simulink model "Energy"  (R2024b)
settings: Solver=ode1  StartTime=0.0  StopTime=955800  FixedStep=1  RelTol=1e-3
(part 2 of 3)

== matlab function Energy/工况生成器 ==
  data: t input; P_out output
function P_out = fcn(t)
%% 工况生成函数2
%% 输入: t - 仿真时间 (s)
%% 输出: P_out - 功率 (kW)

%% ===== 工况数据 =====
% 功率点 (kW)
P_table = [64.039, 57.95, 72.892, 53.239, 371.167, 81.182, 152.606, ...
           55.814, 52.287, 87.468, 57.663, 57.95, 64.502];

% 持续时间 (s) = 小时 × 3600
T_duration = [3, 112, 5, 6, 0.2, 8, 8, 3, 0.3, 1, 4, 112, 3] * 3600;

%% ===== 累计时间断点 =====
T_bp = [0, 10800, 414000, 432000, 453600, 454320, 483120, 511920, ...
        522720, 523800, 527400, 541800, 945000, 955800];

%% ===== 根据时间查找功率 =====
n = 13;
P_out = P_table(n);  % 默认最后一个

for k = 1:n
    if t >= T_bp(k) && t < T_bp(k+1)
        P_out = P_table(k);
        break;
    end
end

end

== matlab function Energy/Subsystem6/DCDC1_2 ==
  data: V_out input; I_in input; V_in input; I_out output
function I_out = fcn(V_out,I_in, V_in)
%% DCDC模型 - 输入电流计算输出电流
%% 输入:
%%   I_in  - 输入电流 (A)
%%   V_in  - 输入电压 (V)
%%   V_out - 输出电压 (V)
%% 输出:
%%   I_out - 输出电流 (A)

%% ===== 效率MAP表 =====
% 输入电压断点 (V)
V_bp = [160, 180, 200, 220, 240, 260, 280];

% 输入电流断点 (A)
I_bp = [0, 20, 40, 60, 80, 100, 120, 140, 160, 180, 200];

% 效率表 (%)，行=电流，列=电压
Eta_map = [
    86, 86, 86, 86, 86, 86, 86;
    88, 88, 87, 87, 87, 87, 86;
    92, 91, 91, 90, 89, 88, 87;
    94, 93, 93, 92, 91, 90, 88;
    94.5, 94, 94, 93, 92, 91, 89;
    95, 94.5, 94, 93.5, 93, 91, 90;
    95, 94.5, 94.5, 94, 93, 92, 91;
    95, 95, 94.5, 94, 93.5, 93, 91;
    95, 95, 94.5, 94, 93, 92, 91;
    95, 94.5, 94.5, 93, 92, 91, 91;
    95, 94.5, 94, 92, 91, 91, 91
] / 100;

%% ===== 输入限幅 =====
V_in_clamp = max(160, min(280, V_in));
I_in_clamp = max(0, min(200, I_in));

%% ===== 查表获取效率 =====
% 找电压区间
nV = 7;
jV = 1;
for j = 1:nV-1
    if V_in_clamp >= V_bp(j) && V_in_clamp <= V_bp(j+1)
        jV = j;
        break;
    end
end
if V_in_clamp >= V_bp(nV)
    jV = nV - 1;
end
tV = (V_in_clamp - V_bp(jV)) / (V_bp(jV+1) - V_bp(jV));

% 找电流区间
nI = 11;
iI = 1;
for i = 1:nI-1
    if I_in_clamp >= I_bp(i) && I_in_clamp <= I_bp(i+1)
        iI = i;
        break;
    end
end
if I_in_clamp >= I_bp(nI)
    iI = nI - 1;
end
tI = (I_in_clamp - I_bp(iI)) / (I_bp(iI+1) - I_bp(iI));

% 双线性插值
eta_11 = Eta_map(iI, jV);
eta_12 = Eta_map(iI, jV+1);
eta_21 = Eta_map(iI+1, jV);
eta_22 = Eta_map(iI+1, jV+1);

eta_1 = eta_11 + tV * (eta_12 - eta_11);
eta_2 = eta_21 + tV * (eta_22 - eta_21);
eta = eta_1 + tI * (eta_2 - eta_1);

%% ===== 计算输出电流 =====
P_in = V_in * I_in;
P_out = P_in * eta;
V_out_safe = max(V_out, 1);
I_out = P_out / V_out_safe;

end

== matlab function Energy/Subsystem/目标输出功率 ==
  data: P_target input; dt input; P_out output
function P_out = fcn(P_target, dt)
%% 燃料电池预热控制器 - 带热机跳过功能
%% 输入:
%%   P_target - 目标功率 (kW)
%%   dt       - 采样时间 (s)
%% 输出:
%%   P_out    - 输出功率 (kW)

%% ===== 参数设置 =====
T_warmup = 1800;       % 预热时间 30分钟
P_warmup = 5;          % 预热功率上限 5kW
T_hot_keep = 18000;    % 热机保持时间 5小时 = 5*3600s

%% ===== 状态变量 =====
persistent timer_run timer_stop is_running is_hot
if isempty(timer_run)
    timer_run = 0;      % 运行计时器
    timer_stop = 0;     % 停机计时器
    is_running = 0;     % 运行状态
    is_hot = 0;         % 热机状态：0=冷机，1=已热机
end

%% ===== 状态机逻辑 =====
if P_target > 0
    % 启动/运行中
    if is_running == 0
        % 刚启动
        is_running = 1;
        timer_run = 0;
        
        % 判断是否需要热机
        if is_hot == 1 && timer_stop <= T_hot_keep
            % 停机5小时内，跳过热机
            timer_run = T_warmup + 1;  % 直接跳过热机阶段
        else
            % 冷机或停机超过5小时，需要热机
            timer_run = 0;
        end
    end
    
    timer_run = timer_run + dt;
    timer_stop = 0;  % 清空停机计时
    
    % 完成热机后标记
    if timer_run > T_warmup
        is_hot = 1;
    end
else
    % 停机
    if is_running == 1
        % 刚停机
        is_running = 0;
        timer_stop = 0;
    end
    
    timer_stop = timer_stop + dt;
    timer_run = 0;
    
    % 停机超过5小时，热机状态清除
    if timer_stop > T_hot_keep
        is_hot = 0;
    end
end

%% ===== 功率选择 =====
if P_target <= 0
    P_out = 0;
elseif timer_run <= T_warmup
    % 热机阶段，限制最大5kW
    P_out = min(P_target, P_warmup);
else
    % 热机完成，输出等于输入
    P_out = P_target;
end

end

== matlab function Energy/Subsystem/DCDC1_1 ==
  data: P_out input; V_out input; I_out output; V_in input; I_in output
function [I_out, I_in] = fcn(P_out, V_out, V_in)
%% DCDC模型 - 输出功率反算输入电流
%% 输入:
%%   P_out - 输出功率 (W)
%%   V_out - 输出电压 (V)
%%   V_in  - 输入电压 (V)
%% 输出:
%%   I_out - 输出电流 (A)
%%   I_in  - 输入电流 (A)

%% ===== 效率MAP表 =====
% 输入电压断点 (V)
V_bp = [160, 180, 200, 220, 240, 260, 280];

% 输入电流断点 (A)
I_bp = [0, 20, 40, 60, 80, 100, 120, 140, 160, 180, 200];

% 效率表 (%)，行=电流，列=电压
Eta_map = [
    86, 86, 86, 86, 86, 86, 86;
    88, 88, 87, 87, 87, 87, 86;
    92, 91, 91, 90, 89, 88, 87;
    94, 93, 93, 92, 91, 90, 88;
    94.5, 94, 94, 93, 92, 91, 89;
    95, 94.5, 94, 93.5, 93, 91, 90;
    95, 94.5, 94.5, 94, 93, 92, 91;
    95, 95, 94.5, 94, 93.5, 93, 91;
    95, 95, 94.5, 94, 93, 92, 91;
    95, 94.5, 94.5, 93, 92, 91, 91;
    95, 94.5, 94, 92, 91, 91, 91
] / 100;

%% ===== 输出电流（直接计算） =====
V_out_safe = max(V_out, 1);
I_out = 1000*P_out / V_out_safe;

%% ===== 迭代求输入电流 =====
V_in_clamp = max(160, min(280, V_in));
V_in_safe = max(V_in, 1);

% 初始估计效率
eta = 0.94;

% 迭代3次足够收敛
for iter = 1:3
    % 根据效率计算输入功率和电流
    P_in = 1000*P_out / eta;
    I_in_est = P_in / V_in_safe;
    I_in_clamp = max(0, min(200, I_in_est));
    
    % 查表获取新效率
    eta = lookup_eta(V_in_clamp, I_in_clamp, V_bp, I_bp, Eta_map);
end

%% ===== 最终输入电流 =====
P_in = 1000*P_out / eta;
I_in = P_in / V_in_safe;

end

%% ===== 效率查表函数 =====
function eta = lookup_eta(V_in, I_in, V_bp, I_bp, Eta_map)
    % 找电压区间
    nV = 7;
    jV = 1;
    for j = 1:nV-1
        if V_in >= V_bp(j) && V_in <= V_bp(j+1)
            jV = j;
            break;
        end
    end
    if V_in >= V_bp(nV)
        jV = nV - 1;
    end
    tV = (V_in - V_bp(jV)) / (V_bp(jV+1) - V_bp(jV));
    
    % 找电流区间
    nI = 11;
    iI = 1;
    for i = 1:nI-1
        if I_in >= I_bp(i) && I_in <= I_bp(i+1)
            iI = i;
            break;
        end
    end
    if I_in >= I_bp(nI)
        iI = nI - 1;
    end
    tI = (I_in - I_bp(iI)) / (I_bp(iI+1) - I_bp(iI));
    
    % 双线性插值
    eta_11 = Eta_map(iI, jV);
    eta_12 = Eta_map(iI, jV+1);
    eta_21 = Eta_map(iI+1, jV);
    eta_22 = Eta_map(iI+1, jV+1);
    
    eta_1 = eta_11 + tV * (eta_12 - eta_11);
    eta_2 = eta_21 + tV * (eta_22 - eta_21);
    eta = eta_1 + tI * (eta_2 - eta_1);
end

== matlab function Energy/Subsystem/输出电流加载限制 ==
  data: I_target input; I_current input; I_out output; dt input
function I_out = fcn(I_target,I_current,  dt)
%% 电流斜坡控制器 - 反馈版
%% 输入:
%%   I_current - 当前电流 (A)，从输出反馈
%%   I_target  - 目标电流 (A) 
%%   dt        - 采样时间 (s)
%% 输出:
%%   I_out     - 输出电流 (A)

%% ===== 参数设置 =====
rate_up = 1;    % 上升速率 1A/s
rate_down = 2;  % 下降速率 2A/s

%% ===== 斜坡控制 =====
delta = I_target - I_current;

if delta > 0
    % 目标 > 当前，每秒+1A
    I_out = I_current + rate_up * dt;
    if I_out > I_target
        I_out = I_target;
    end
elseif delta < 0
    % 目标 < 当前，每秒-2A
    I_out = I_current - rate_down * dt;
    if I_out < I_target
        I_out = I_target;
    end
else
    I_out = I_current;
end

%% ===== 输出限幅 =====
I_out = max(0, I_out);

end

== matlab function Energy/Subsystem/DCDC1_2 ==
  data: V_out input; I_in input; V_in input; I_out output
function I_out = fcn(V_out,I_in, V_in)
%% DCDC模型 - 输入电流计算输出电流
%% 输入:
%%   I_in  - 输入电流 (A)
%%   V_in  - 输入电压 (V)
%%   V_out - 输出电压 (V)
%% 输出:
%%   I_out - 输出电流 (A)

%% ===== 效率MAP表 =====
% 输入电压断点 (V)
V_bp = [160, 180, 200, 220, 240, 260, 280];

% 输入电流断点 (A)
I_bp = [0, 20, 40, 60, 80, 100, 120, 140, 160, 180, 200];

% 效率表 (%)，行=电流，列=电压
Eta_map = [
    86, 86, 86, 86, 86, 86, 86;
    88, 88, 87, 87, 87, 87, 86;
    92, 91, 91, 90, 89, 88, 87;
    94, 93, 93, 92, 91, 90, 88;
    94.5, 94, 94, 93, 92, 91, 89;
    95, 94.5, 94, 93.5, 93, 91, 90;
    95, 94.5, 94.5, 94, 93, 92, 91;
    95, 95, 94.5, 94, 93.5, 93, 91;
    95, 95, 94.5, 94, 93, 92, 91;
    95, 94.5, 94.5, 93, 92, 91, 91;
    95, 94.5, 94, 92, 91, 91, 91
] / 100;

%% ===== 输入限幅 =====
V_in_clamp = max(160, min(280, V_in));
I_in_clamp = max(0, min(200, I_in));

%% ===== 查表获取效率 =====
% 找电压区间
nV = 7;
jV = 1;
for j = 1:nV-1
    if V_in_clamp >= V_bp(j) && V_in_clamp <= V_bp(j+1)
        jV = j;
        break;
    end
end
if V_in_clamp >= V_bp(nV)
    jV = nV - 1;
end
tV = (V_in_clamp - V_bp(jV)) / (V_bp(jV+1) - V_bp(jV));

% 找电流区间
nI = 11;
iI = 1;
for i = 1:nI-1
    if I_in_clamp >= I_bp(i) && I_in_clamp <= I_bp(i+1)
        iI = i;
        break;
    end
end
if I_in_clamp >= I_bp(nI)
    iI = nI - 1;
end
tI = (I_in_clamp - I_bp(iI)) / (I_bp(iI+1) - I_bp(iI));

% 双线性插值
eta_11 = Eta_map(iI, jV);
eta_12 = Eta_map(iI, jV+1);
eta_21 = Eta_map(iI+1, jV);
eta_22 = Eta_map(iI+1, jV+1);

eta_1 = eta_11 + tV * (eta_12 - eta_11);
eta_2 = eta_21 + tV * (eta_22 - eta_21);
eta = eta_1 + tI * (eta_2 - eta_1);

%% ===== 计算输出电流 =====
P_in = V_in * I_in;
P_out = P_in * eta;
V_out_safe = max(V_out, 1);
I_out = P_out / V_out_safe;

end

== matlab function Energy/Subsystem6/目标输出功率 ==
  data: P_target input; dt input; P_out output
function P_out = fcn(P_target, dt)
%% 燃料电池预热控制器 - 带热机跳过功能
%% 输入:
%%   P_target - 目标功率 (kW)
%%   dt       - 采样时间 (s)
%% 输出:
%%   P_out    - 输出功率 (kW)

%% ===== 参数设置 =====
T_warmup = 1800;       % 预热时间 30分钟
P_warmup = 5;          % 预热功率上限 5kW
T_hot_keep = 18000;    % 热机保持时间 5小时 = 5*3600s

%% ===== 状态变量 =====
persistent timer_run timer_stop is_running is_hot
if isempty(timer_run)
    timer_run = 0;      % 运行计时器
    timer_stop = 0;     % 停机计时器
    is_running = 0;     % 运行状态
    is_hot = 0;         % 热机状态：0=冷机，1=已热机
end

%% ===== 状态机逻辑 =====
if P_target > 0
    % 启动/运行中
    if is_running == 0
        % 刚启动
        is_running = 1;
        timer_run = 0;
        
        % 判断是否需要热机
        if is_hot == 1 && timer_stop <= T_hot_keep
            % 停机5小时内，跳过热机
            timer_run = T_warmup + 1;  % 直接跳过热机阶段
        else
            % 冷机或停机超过5小时，需要热机
            timer_run = 0;
        end
    end
    
    timer_run = timer_run + dt;
    timer_stop = 0;  % 清空停机计时
    
    % 完成热机后标记
    if timer_run > T_warmup
        is_hot = 1;
    end
else
    % 停机
    if is_running == 1
        % 刚停机
        is_running = 0;
        timer_stop = 0;
    end
    
    timer_stop = timer_stop + dt;
    timer_run = 0;
    
    % 停机超过5小时，热机状态清除
    if timer_stop > T_hot_keep
        is_hot = 0;
    end
end

%% ===== 功率选择 =====
if P_target <= 0
    P_out = 0;
elseif timer_run <= T_warmup
    % 热机阶段，限制最大5kW
    P_out = min(P_target, P_warmup);
else
    % 热机完成，输出等于输入
    P_out = P_target;
end

end

== matlab function Energy/240kW功率分配 ==
  data: V_battery input; SOC input; P_battery input; P1 output; P2 output; P3 output; P4 output; P5 output; P6 output; P7 output; P8 output; P_fuelcell input; dt input
function [P1, P2, P3, P4, P5, P6, P7, P8] = fcn(V_battery, SOC, P_battery, P_fuelcell, dt)
%% 能量管理控制器 - 不停机策略
%% 挡位: 0(仅P_load=0), 50, 65, 85, 120 kW
%% 
%% 核心规则：
%% 1. 只有P_load=0才允许停机，否则至少保持1档运行
%% 2. SOC硬保护：0.5-0.9，超限立即响应
%% 3. 正常模式：滞回切换 + 冷却时间

%% ===== SOC硬保护阈值 =====
SOC_max = 0.9;
SOC_min = 0.5;
SOC_discharge_stop = 0.65;
SOC_charge_stop = 0.7;

%% ===== 挡位功率 (kW) =====
% 0档=0, 1档=50, 2档=65, 3档=85, 4档=120
Gear_power = [0, 50, 65, 85, 120];

%% ===== 挡位切换阈值 (kW) =====
% 主力挡位2档(65kW)覆盖55-75kW
Gear_up = [1, 55, 75, 100];       % 0→1, 1→2, 2→3, 3→4
Gear_down = [0, 48, 68, 88];      % 1→0(仅P=0), 2→1, 3→2, 4→3

%% ===== 冷却时间 =====
T_cooldown = 120;

%% ===== 过载阈值 =====
P_overload = 150;

%% ===== 状态变量 =====
persistent gear_state discharge_mode charge_mode cooldown_timer
if isempty(gear_state)
    gear_state = 2;  % 初始65kW挡
    discharge_mode = 0;
    charge_mode = 0;
    cooldown_timer = 0;
end

%% ===== 更新冷却计时器 =====
if cooldown_timer > 0
    cooldown_timer = cooldown_timer - dt;
end

%% ===== 计算负载功率 (kW) =====
P_load = P_fuelcell + P_battery;
P_load = max(0, P_load);

%% ===== 停机判断：仅当P_load=0 =====
if P_load < 0.1
    % 完全无负载才停机
    gear_state = 0;
    P1 = 0; P2 = 0; P3 = 0; P4 = 0;
    P5 = 0; P6 = 0; P7 = 0; P8 = 0;
    
elseif P_load > P_overload
    %% ===== 过载保护 =====
    gear_state = 4;
    P1 = 30; P2 = 30; P3 = 30; P4 = 30;
    P5 = 0; P6 = 0; P7 = 0; P8 = 0;
    
else
    %% ===== 从停机恢复 =====
    if gear_state == 0
        gear_state = 2;  % 恢复到主力档位
        cooldown_timer = T_cooldown;
    end
    
    %% ===== SOC保护模式滞回更新 =====
    if SOC > SOC_max
        discharge_mode = 1;
    elseif SOC <= SOC_discharge_stop
        discharge_mode = 0;
    end
    
    if SOC < SOC_min
        charge_mode = 1;
    elseif SOC >= SOC_charge_stop
        charge_mode = 0;
    end
    
    %% ===== SOC硬保护（立即响应）=====
    if discharge_mode == 1
        % SOC > 0.9：降档让电池放电
        if P_battery <= 0
            gear_state = gear_state - 1;
            % 最低降到1档，不停机！
            if gear_state < 1
                gear_state = 1;
            end
        end
        
    elseif charge_mode == 1
        % SOC < 0.5：升档让电池充电
        if P_battery >= 0
            gear_state = gear_state + 1;
            if gear_state > 4
                gear_state = 4;
            end
        end
        
    else
        %% ===== 正常模式：滞回切换 =====
        if cooldown_timer <= 0
            need_change = 0;
            
            % 注意：不会降到0档（除非P_load=0已在前面处理）
            if gear_state == 1
                if P_load > Gear_up(2)
                    gear_state = 2;
                    need_change = 1;
                end
            elseif gear_state == 2
                if P_load < Gear_down(2)
                    gear_state = 1;
                    need_change = 1;
                elseif P_load > Gear_up(3)
                    gear_state = 3;
                    need_change = 1;
                end
            elseif gear_state == 3
                if P_load < Gear_down(3)
                    gear_state = 2;
                    need_change = 1;
                elseif P_load > Gear_up(4)
                    gear_state = 4;
                    need_change = 1;
                end
            elseif gear_state == 4
                if P_load < Gear_down(4)
                    gear_state = 3;
                    need_change = 1;
                end
            end
            
            if need_change == 1
                cooldown_timer = T_cooldown;
            end
        end
    end
    
    %% ===== 按挡位分配功率 =====
    if gear_state == 1
        P1 = 12.5; P2 = 12.5; P3 = 12.5; P4 = 12.5;  % 50kW
    elseif gear_state == 2
        P1 = 16.25; P2 = 16.25; P3 = 16.25; P4 = 16.25;  % 65kW
    elseif gear_state == 3
        P1 = 21.25; P2 = 21.25; P3 = 21.25; P4 = 21.25;  % 85kW
    else
        P1 = 30; P2 = 30; P3 = 30; P4 = 30;  % 120kW
    end
    P5 = 0; P6 = 0; P7 = 0; P8 = 0;
end

end

== matlab function Energy/Subsystem6/输出电流加载限制 ==
  data: I_target input; I_current input; I_out output; dt input
function I_out = fcn(I_target,I_current,  dt)
%% 电流斜坡控制器 - 反馈版
%% 输入:
%%   I_current - 当前电流 (A)，从输出反馈
%%   I_target  - 目标电流 (A) 
%%   dt        - 采样时间 (s)
%% 输出:
%%   I_out     - 输出电流 (A)

%% ===== 参数设置 =====
rate_up = 1;    % 上升速率 1A/s
rate_down = 2;  % 下降速率 2A/s

%% ===== 斜坡控制 =====
delta = I_target - I_current;

if delta > 0
    % 目标 > 当前，每秒+1A
    I_out = I_current + rate_up * dt;
    if I_out > I_target
        I_out = I_target;
    end
elseif delta < 0
    % 目标 < 当前，每秒-2A
    I_out = I_current - rate_down * dt;
    if I_out < I_target
        I_out = I_target;
    end
else
    I_out = I_current;
end

%% ===== 输出限幅 =====
I_out = max(0, I_out);

end

== matlab function Energy/Subsystem7/32kW燃料电池 ==
  data: I_in input; V output
function V = fcn(I_in)
%% 燃料电池模型 - 极化曲线
%% 输入: I_in - 输入电流 (A)
%% 输出: V    - 输出电压 (V)

%% ===== 极化曲线数据 =====
I_table = [0, 16.77, 31.67, 48.13, 64.92, 80.76, 98.06, 115.48, 132.58, 150.51, 170.44, 186.07];
V_table = [248.1, 218.42, 212.82, 207.8, 205, 202.68, 200, 197.8, 196.44, 194.26, 192.66, 191.2];

%% ===== 电流限幅 =====
I_max = 186.07;
I = max(0, min(I_in, I_max));

%% ===== 根据电流查找电压 =====
V = V_table(1);  % 初始化
n = 12;

for k = 1:n-1
    if I >= I_table(k) && I <= I_table(k+1)
        t = (I - I_table(k)) / (I_table(k+1) - I_table(k));
        V = V_table(k) + t * (V_table(k+1) - V_table(k));
        break;
    end
end

if I >= I_table(n)
    V = V_table(n);
end

end

== matlab function Energy/Subsystem/32kW燃料电池 ==
  data: I_in input; V output
function V = fcn(I_in)
%% 燃料电池模型 - 极化曲线
%% 输入: I_in - 输入电流 (A)
%% 输出: V    - 输出电压 (V)

%% ===== 极化曲线数据 =====
I_table = [0, 16.77, 31.67, 48.13, 64.92, 80.76, 98.06, 115.48, 132.58, 150.51, 170.44, 186.07];
V_table = [248.1, 218.42, 212.82, 207.8, 205, 202.68, 200, 197.8, 196.44, 194.26, 192.66, 191.2];

%% ===== 电流限幅 =====
I_max = 186.07;
I = max(0, min(I_in, I_max));

%% ===== 根据电流查找电压 =====
V = V_table(1);  % 初始化
n = 12;

for k = 1:n-1
    if I >= I_table(k) && I <= I_table(k+1)
        t = (I - I_table(k)) / (I_table(k+1) - I_table(k));
        V = V_table(k) + t * (V_table(k+1) - V_table(k));
        break;
    end
end

if I >= I_table(n)
    V = V_table(n);
end

end

== matlab function Energy/Subsystem7/DCDC1_1 ==
  data: P_out input; V_out input; I_out output; V_in input; I_in output
function [I_out, I_in] = fcn(P_out, V_out, V_in)
%% DCDC模型 - 输出功率反算输入电流
%% 输入:
%%   P_out - 输出功率 (W)
%%   V_out - 输出电压 (V)
%%   V_in  - 输入电压 (V)
%% 输出:
%%   I_out - 输出电流 (A)
%%   I_in  - 输入电流 (A)

%% ===== 效率MAP表 =====
% 输入电压断点 (V)
V_bp = [160, 180, 200, 220, 240, 260, 280];

% 输入电流断点 (A)
I_bp = [0, 20, 40, 60, 80, 100, 120, 140, 160, 180, 200];

% 效率表 (%)，行=电流，列=电压
Eta_map = [
    86, 86, 86, 86, 86, 86, 86;
    88, 88, 87, 87, 87, 87, 86;
    92, 91, 91, 90, 89, 88, 87;
    94, 93, 93, 92, 91, 90, 88;
    94.5, 94, 94, 93, 92, 91, 89;
    95, 94.5, 94, 93.5, 93, 91, 90;
    95, 94.5, 94.5, 94, 93, 92, 91;
    95, 95, 94.5, 94, 93.5, 93, 91;
    95, 95, 94.5, 94, 93, 92, 91;
    95, 94.5, 94.5, 93, 92, 91, 91;
    95, 94.5, 94, 92, 91, 91, 91
] / 100;

%% ===== 输出电流（直接计算） =====
V_out_safe = max(V_out, 1);
I_out = 1000*P_out / V_out_safe;

%% ===== 迭代求输入电流 =====
V_in_clamp = max(160, min(280, V_in));
V_in_safe = max(V_in, 1);

% 初始估计效率
eta = 0.94;

% 迭代3次足够收敛
for iter = 1:3
    % 根据效率计算输入功率和电流
    P_in = 1000*P_out / eta;
    I_in_est = P_in / V_in_safe;
    I_in_clamp = max(0, min(200, I_in_est));
    
    % 查表获取新效率
    eta = lookup_eta(V_in_clamp, I_in_clamp, V_bp, I_bp, Eta_map);
end

%% ===== 最终输入电流 =====
P_in = 1000*P_out / eta;
I_in = P_in / V_in_safe;

end

%% ===== 效率查表函数 =====
function eta = lookup_eta(V_in, I_in, V_bp, I_bp, Eta_map)
    % 找电压区间
    nV = 7;
    jV = 1;
    for j = 1:nV-1
        if V_in >= V_bp(j) && V_in <= V_bp(j+1)
            jV = j;
            break;
        end
    end
    if V_in >= V_bp(nV)
        jV = nV - 1;
    end
    tV = (V_in - V_bp(jV)) / (V_bp(jV+1) - V_bp(jV));
    
    % 找电流区间
    nI = 11;
    iI = 1;
    for i = 1:nI-1
        if I_in >= I_bp(i) && I_in <= I_bp(i+1)
            iI = i;
            break;
        end
    end
    if I_in >= I_bp(nI)
        iI = nI - 1;
    end
    tI = (I_in - I_bp(iI)) / (I_bp(iI+1) - I_bp(iI));
    
    % 双线性插值
    eta_11 = Eta_map(iI, jV);
    eta_12 = Eta_map(iI, jV+1);
    eta_21 = Eta_map(iI+1, jV);
    eta_22 = Eta_map(iI+1, jV+1);
    
    eta_1 = eta_11 + tV * (eta_12 - eta_11);
    eta_2 = eta_21 + tV * (eta_22 - eta_21);
    eta = eta_1 + tI * (eta_2 - eta_1);
end

== matlab function Energy/Subsystem7/DCDC1_2 ==
  data: V_out input; I_in input; V_in input; I_out output
function I_out = fcn(V_out,I_in, V_in)
%% DCDC模型 - 输入电流计算输出电流
%% 输入:
%%   I_in  - 输入电流 (A)
%%   V_in  - 输入电压 (V)
%%   V_out - 输出电压 (V)
%% 输出:
%%   I_out - 输出电流 (A)

%% ===== 效率MAP表 =====
% 输入电压断点 (V)
V_bp = [160, 180, 200, 220, 240, 260, 280];

% 输入电流断点 (A)
I_bp = [0, 20, 40, 60, 80, 100, 120, 140, 160, 180, 200];

% 效率表 (%)，行=电流，列=电压
Eta_map = [
    86, 86, 86, 86, 86, 86, 86;
    88, 88, 87, 87, 87, 87, 86;
    92, 91, 91, 90, 89, 88, 87;
    94, 93, 93, 92, 91, 90, 88;
    94.5, 94, 94, 93, 92, 91, 89;
    95, 94.5, 94, 93.5, 93, 91, 90;
    95, 94.5, 94.5, 94, 93, 92, 91;
    95, 95, 94.5, 94, 93.5, 93, 91;
    95, 95, 94.5, 94, 93, 92, 91;
    95, 94.5, 94.5, 93, 92, 91, 91;
    95, 94.5, 94, 92, 91, 91, 91
] / 100;

%% ===== 输入限幅 =====
V_in_clamp = max(160, min(280, V_in));
I_in_clamp = max(0, min(200, I_in));

%% ===== 查表获取效率 =====
% 找电压区间
nV = 7;
jV = 1;
for j = 1:nV-1
    if V_in_clamp >= V_bp(j) && V_in_clamp <= V_bp(j+1)
        jV = j;
        break;
    end
end
if V_in_clamp >= V_bp(nV)
    jV = nV - 1;
end
tV = (V_in_clamp - V_bp(jV)) / (V_bp(jV+1) - V_bp(jV));

% 找电流区间
nI = 11;
iI = 1;
for i = 1:nI-1
    if I_in_clamp >= I_bp(i) && I_in_clamp <= I_bp(i+1)
        iI = i;
        break;
    end
end
if I_in_clamp >= I_bp(nI)
    iI = nI - 1;
end
tI = (I_in_clamp - I_bp(iI)) / (I_bp(iI+1) - I_bp(iI));

% 双线性插值
eta_11 = Eta_map(iI, jV);
eta_12 = Eta_map(iI, jV+1);
eta_21 = Eta_map(iI+1, jV);
eta_22 = Eta_map(iI+1, jV+1);

eta_1 = eta_11 + tV * (eta_12 - eta_11);
eta_2 = eta_21 + tV * (eta_22 - eta_21);
eta = eta_1 + tI * (eta_2 - eta_1);

%% ===== 计算输出电流 =====
P_in = V_in * I_in;
P_out = P_in * eta;
V_out_safe = max(V_out, 1);
I_out = P_out / V_out_safe;

end

== matlab function Energy/Subsystem7/目标输出功率 ==
  data: P_target input; dt input; P_out output
function P_out = fcn(P_target, dt)
%% 燃料电池预热控制器 - 带热机跳过功能
%% 输入:
%%   P_target - 目标功率 (kW)
%%   dt       - 采样时间 (s)
%% 输出:
%%   P_out    - 输出功率 (kW)

%% ===== 参数设置 =====
T_warmup = 1800;       % 预热时间 30分钟
P_warmup = 5;          % 预热功率上限 5kW
T_hot_keep = 18000;    % 热机保持时间 5小时 = 5*3600s

%% ===== 状态变量 =====
persistent timer_run timer_stop is_running is_hot
if isempty(timer_run)
    timer_run = 0;      % 运行计时器
    timer_stop = 0;     % 停机计时器
    is_running = 0;     % 运行状态
    is_hot = 0;         % 热机状态：0=冷机，1=已热机
end

%% ===== 状态机逻辑 =====
if P_target > 0
    % 启动/运行中
    if is_running == 0
        % 刚启动
        is_running = 1;
        timer_run = 0;
        
        % 判断是否需要热机
        if is_hot == 1 && timer_stop <= T_hot_keep
            % 停机5小时内，跳过热机
            timer_run = T_warmup + 1;  % 直接跳过热机阶段
        else
            % 冷机或停机超过5小时，需要热机
            timer_run = 0;
        end
    end
    
    timer_run = timer_run + dt;
    timer_stop = 0;  % 清空停机计时
    
    % 完成热机后标记
    if timer_run > T_warmup
        is_hot = 1;
    end
else
    % 停机
    if is_running == 1
        % 刚停机
        is_running = 0;
        timer_stop = 0;
    end
    
    timer_stop = timer_stop + dt;
    timer_run = 0;
    
    % 停机超过5小时，热机状态清除
    if timer_stop > T_hot_keep
        is_hot = 0;
    end
end

%% ===== 功率选择 =====
if P_target <= 0
    P_out = 0;
elseif timer_run <= T_warmup
    % 热机阶段，限制最大5kW
    P_out = min(P_target, P_warmup);
else
    % 热机完成，输出等于输入
    P_out = P_target;
end

end

== matlab function Energy/Subsystem7/输出电流加载限制 ==
  data: I_target input; I_current input; I_out output; dt input
function I_out = fcn(I_target,I_current,  dt)
%% 电流斜坡控制器 - 反馈版
%% 输入:
%%   I_current - 当前电流 (A)，从输出反馈
%%   I_target  - 目标电流 (A) 
%%   dt        - 采样时间 (s)
%% 输出:
%%   I_out     - 输出电流 (A)

%% ===== 参数设置 =====
rate_up = 1;    % 上升速率 1A/s
rate_down = 2;  % 下降速率 2A/s

%% ===== 斜坡控制 =====
delta = I_target - I_current;

if delta > 0
    % 目标 > 当前，每秒+1A
    I_out = I_current + rate_up * dt;
    if I_out > I_target
        I_out = I_target;
    end
elseif delta < 0
    % 目标 < 当前，每秒-2A
    I_out = I_current - rate_down * dt;
    if I_out < I_target
        I_out = I_target;
    end
else
    I_out = I_current;
end

%% ===== 输出限幅 =====
I_out = max(0, I_out);

end

== matlab function Energy/240kW功率分配-跟随-不响应370kW ==
  data: V_battery input; SOC input; P_battery input; P1 output; P2 output; P3 output; P4 output; P5 output; P6 output; P7 output; P8 output; P_fuelcell input
function [P1, P2, P3, P4, P5, P6, P7, P8] = fcn(V_battery, SOC, P_battery, P_fuelcell)
%% 能量管理控制器 - 功率分配
%% 输入:
%%   SOC        - 蓄电池荷电状态 (0~1)
%%   P_battery  - 蓄电池功率 (kW)
%%   P_fuelcell - 燃料电池功率 (kW)
%%   V_battery  - 蓄电池电压 (V)
%% 输出:
%%   P1~P8      - 8个通道功率分配 (kW)

%% ===== SOC阈值设置 =====
SOC_charge_start = 0.5;
SOC_charge_stop = 0.7;
SOC_discharge_start = 0.8;
SOC_discharge_stop = 0.6;

%% ===== 功率分配阈值 (kW) =====
P_low = 120;
P_high = 180;
P_overload = 300;     % 过载阈值
P_max_each = 32;      % 每通道最大32kW
P_min_each = 5;       % 每通道最小5kW

%% ===== 充放电电流 =====
I_charge = 100;

%% ===== 滞回控制状态 =====
persistent charge_mode discharge_mode
if isempty(charge_mode)
    charge_mode = 0;
    discharge_mode = 0;
end

%% ===== SOC滞回控制逻辑 =====
if SOC < SOC_charge_start
    charge_mode = 1;
elseif SOC >= SOC_charge_stop
    charge_mode = 0;
end

if SOC > SOC_discharge_start
    discharge_mode = 1;
elseif SOC <= SOC_discharge_stop
    discharge_mode = 0;
end

%% ===== 计算系统需求功率 (kW) =====
P_base = P_fuelcell + P_battery;

if charge_mode == 1
    P_demand = P_base + V_battery * I_charge / 1000;
elseif discharge_mode == 1
    P_demand = P_base - V_battery * I_charge / 1000;
else
    P_demand = P_base;
end

P_demand = max(0, P_demand);

%% ===== 过载保护：P_base > 300kW =====
if P_base > P_overload
    % 前4通道满功率32kW，后4通道关闭
    P1 = P_max_each; P2 = P_max_each; P3 = P_max_each; P4 = P_max_each;
    P5 = 0; P6 = 0; P7 = 0; P8 = 0;
else
    %% ===== 正常功率分配 =====
    if P_demand <= P_low
        P_each = P_demand / 4;
        P1 = P_each; P2 = P_each; P3 = P_each; P4 = P_each;
        P5 = 0; P6 = 0; P7 = 0; P8 = 0;
    elseif P_demand > P_high
        P_each = P_demand / 8;
        P1 = P_each; P2 = P_each; P3 = P_each; P4 = P_each;
        P5 = P_each; P6 = P_each; P7 = P_each; P8 = P_each;
    else
        P_each = P_demand / 4;
        P1 = P_each; P2 = P_each; P3 = P_each; P4 = P_each;
        P5 = 0; P6 = 0; P7 = 0; P8 = 0;
    end
    
    %% ===== 每通道限幅：最大32kW =====
    P1 = min(P1, P_max_each);
    P2 = min(P2, P_max_each);
    P3 = min(P3, P_max_each);
    P4 = min(P4, P_max_each);
    P5 = min(P5, P_max_each);
    P6 = min(P6, P_max_each);
    P7 = min(P7, P_max_each);
    P8 = min(P8, P_max_each);
    
    %% ===== 每通道最小阈值：小于5kW则关闭 =====
    if P1 < P_min_each, P1 = 0; end
    if P2 < P_min_each, P2 = 0; end
    if P3 < P_min_each, P3 = 0; end
    if P4 < P_min_each, P4 = 0; end
    if P5 < P_min_each, P5 = 0; end
    if P6 < P_min_each, P6 = 0; end
    if P7 < P_min_each, P7 = 0; end
    if P8 < P_min_each, P8 = 0; end
end

end

== matlab function Energy/240kW功率分配-跟随-响应370kW ==
  data: V_battery input; SOC input; P_battery input; P1 output; P2 output; P3 output; P4 output; P5 output; P6 output; P7 output; P8 output; P_fuelcell input
function [P1, P2, P3, P4, P5, P6, P7, P8] = fcn(V_battery, SOC, P_battery, P_fuelcell)
%% 能量管理控制器 - 功率分配
%% 输入:
%%   SOC        - 蓄电池荷电状态 (0~1)
%%   P_battery  - 蓄电池功率 (W)
%%   P_fuelcell - 燃料电池功率 (W)
%%   V_battery  - 蓄电池电压 (V)
%% 输出:
%%   P1~P8      - 8个通道功率分配 (kW)

%% ===== SOC阈值设置 =====
SOC_charge_start = 0.5;
SOC_charge_stop = 0.7;
SOC_discharge_start = 0.8;
SOC_discharge_stop = 0.6;

%% ===== 功率分配阈值 (kW) =====
P_low = 120;
P_high = 140;
P_max_each = 32;  % 每通道最大32kW
P_min_each = 5;   % 每通道最小5kW，低于则关闭

%% ===== 充放电电流 =====
I_charge = 100;

%% ===== 滞回控制状态 =====
persistent charge_mode discharge_mode
if isempty(charge_mode)
    charge_mode = 0;
    discharge_mode = 0;
end

%% ===== SOC滞回控制逻辑 =====
if SOC < SOC_charge_start
    charge_mode = 1;
elseif SOC >= SOC_charge_stop
    charge_mode = 0;
end

if SOC > SOC_discharge_start
    discharge_mode = 1;
elseif SOC <= SOC_discharge_stop
    discharge_mode = 0;
end

%% ===== 计算系统需求功率 (kW) =====
P_base = P_fuelcell + P_battery;

if charge_mode == 1
    P_demand = P_base + V_battery * I_charge / 1000;
elseif discharge_mode == 1
    P_demand = P_base - V_battery * I_charge / 1000;
else
    P_demand = P_base;
end

P_demand = max(0, P_demand);

%% ===== 功率分配 =====
if P_demand <= P_low
    P_each = P_demand / 4;
    P1 = P_each; P2 = P_each; P3 = P_each; P4 = P_each;
    P5 = 0; P6 = 0; P7 = 0; P8 = 0;
elseif P_demand > P_high
    P_each = P_demand / 8;
    P1 = P_each; P2 = P_each; P3 = P_each; P4 = P_each;
    P5 = P_each; P6 = P_each; P7 = P_each; P8 = P_each;
else
    P_each = P_demand / 4;
    P1 = P_each; P2 = P_each; P3 = P_each; P4 = P_each;
    P5 = 0; P6 = 0; P7 = 0; P8 = 0;
end

%% ===== 每通道限幅：最大32kW =====
P1 = min(P1, P_max_each);
P2 = min(P2, P_max_each);
P3 = min(P3, P_max_each);
P4 = min(P4, P_max_each);
P5 = min(P5, P_max_each);
P6 = min(P6, P_max_each);
P7 = min(P7, P_max_each);
P8 = min(P8, P_max_each);

%% ===== 每通道最小阈值：小于5kW则关闭 =====
if P1 < P_min_each, P1 = 0; end
if P2 < P_min_each, P2 = 0; end
if P3 < P_min_each, P3 = 0; end
if P4 < P_min_each, P4 = 0; end
if P5 < P_min_each, P5 = 0; end
if P6 < P_min_each, P6 = 0; end
if P7 < P_min_each, P7 = 0; end
if P8 < P_min_each, P8 = 0; end

end

== matlab function Energy/240kW功率分配-5挡位分配32，64，96，128，256 ==
  data: V_battery input; SOC input; P_battery input; P1 output; P2 output; P3 output; P4 output; P5 output; P6 output; P7 output; P8 output; P_fuelcell input; dt input
function [P1, P2, P3, P4, P5, P6, P7, P8] = fcn(V_battery, SOC, P_battery, P_fuelcell, dt)
%% 能量管理控制器 - 不停机策略
%% 挡位: 0(仅P_load=0), 50, 65, 85, 120 kW
%% 
%% 核心规则：
%% 1. 只有P_load=0才允许停机，否则至少保持1档运行
%% 2. SOC硬保护：0.5-0.9，超限立即响应
%% 3. 正常模式：滞回切换 + 冷却时间

%% ===== SOC硬保护阈值 =====
SOC_max = 0.9;
SOC_min = 0.5;
SOC_discharge_stop = 0.65;
SOC_charge_stop = 0.7;

%% ===== 挡位功率 (kW) =====
% 0档=0, 1档=50, 2档=65, 3档=85, 4档=120
Gear_power = [0, 50, 65, 85, 120];

%% ===== 挡位切换阈值 (kW) =====
% 主力挡位2档(65kW)覆盖55-75kW
Gear_up = [1, 55, 75, 100];       % 0→1, 1→2, 2→3, 3→4
Gear_down = [0, 48, 68, 88];      % 1→0(仅P=0), 2→1, 3→2, 4→3

%% ===== 冷却时间 =====
T_cooldown = 120;

%% ===== 过载阈值 =====
P_overload = 150;

%% ===== 状态变量 =====
persistent gear_state discharge_mode charge_mode cooldown_timer
if isempty(gear_state)
    gear_state = 2;  % 初始65kW挡
    discharge_mode = 0;
    charge_mode = 0;
    cooldown_timer = 0;
end

%% ===== 更新冷却计时器 =====
if cooldown_timer > 0
    cooldown_timer = cooldown_timer - dt;
end

%% ===== 计算负载功率 (kW) =====
P_load = P_fuelcell + P_battery;
P_load = max(0, P_load);

%% ===== 停机判断：仅当P_load=0 =====
if P_load < 0.1
    % 完全无负载才停机
    gear_state = 0;
    P1 = 0; P2 = 0; P3 = 0; P4 = 0;
    P5 = 0; P6 = 0; P7 = 0; P8 = 0;
    
elseif P_load > P_overload
    %% ===== 过载保护 =====
    gear_state = 4;
    P1 = 30; P2 = 30; P3 = 30; P4 = 30;
    P5 = 0; P6 = 0; P7 = 0; P8 = 0;
    
else
    %% ===== 从停机恢复 =====
    if gear_state == 0
        gear_state = 2;  % 恢复到主力档位
        cooldown_timer = T_cooldown;
    end
    
    %% ===== SOC保护模式滞回更新 =====
    if SOC > SOC_max
        discharge_mode = 1;
    elseif SOC <= SOC_discharge_stop
        discharge_mode = 0;
    end
    
    if SOC < SOC_min
        charge_mode = 1;
    elseif SOC >= SOC_charge_stop
        charge_mode = 0;
    end
    
    %% ===== SOC硬保护（立即响应）=====
    if discharge_mode == 1
        % SOC > 0.9：降档让电池放电
        if P_battery <= 0
            gear_state = gear_state - 1;
            % 最低降到1档，不停机！
            if gear_state < 1
                gear_state = 1;
            end
        end
        
    elseif charge_mode == 1
        % SOC < 0.5：升档让电池充电
        if P_battery >= 0
            gear_state = gear_state + 1;
            if gear_state > 4
                gear_state = 4;
            end
        end
        
    else
        %% ===== 正常模式：滞回切换 =====
        if cooldown_timer <= 0
            need_change = 0;
            
            % 注意：不会降到0档（除非P_load=0已在前面处理）
            if gear_state == 1
                if P_load > Gear_up(2)
                    gear_state = 2;
                    need_change = 1;
                end
            elseif gear_state == 2
                if P_load < Gear_down(2)
                    gear_state = 1;
                    need_change = 1;
                elseif P_load > Gear_up(3)
                    gear_state = 3;
                    need_change = 1;
                end
            elseif gear_state == 3
                if P_load < Gear_down(3)
                    gear_state = 2;
                    need_change = 1;
                elseif P_load > Gear_up(4)
                    gear_state = 4;
                    need_change = 1;
                end
            elseif gear_state == 4
                if P_load < Gear_down(4)
                    gear_state = 3;
                    need_change = 1;
                end
            end
            
            if need_change == 1
                cooldown_timer = T_cooldown;
            end
        end
    end
    
    %% ===== 按挡位分配功率 =====
    if gear_state == 1
        P1 = 12.5; P2 = 12.5; P3 = 12.5; P4 = 12.5;  % 50kW
    elseif gear_state == 2
        P1 = 16.25; P2 = 16.25; P3 = 16.25; P4 = 16.25;  % 65kW
    elseif gear_state == 3
        P1 = 21.25; P2 = 21.25; P3 = 21.25; P4 = 21.25;  % 85kW
    else
        P1 = 30; P2 = 30; P3 = 30; P4 = 30;  % 120kW
    end
    P5 = 0; P6 = 0; P7 = 0; P8 = 0;
end

end

== matlab function Energy/5kW功率限制 ==
  data: P_target input; dt input; P_out output
function P_out = fcn(P_target, dt)
%% 燃料电池预热控制器 - 功率限制版
%% 输入:
%%   P_target - 目标功率 (W)
%%   dt       - 采样时间 (s)
%% 输出:
%%   P_out    - 输出功率 (W)

%% ===== 参数设置 =====
T_warmup = 1800;    % 预热时间 30分钟
P_warmup = 5;    % 预热功率上限 5kW

%% ===== 状态变量 =====
persistent timer is_running
if isempty(timer)
    timer = 0;
    is_running = 0;
end

%% ===== 计时逻辑 =====
if P_target > 0
    if is_running == 0
        is_running = 1;
        timer = 0;
    end
    timer = timer + dt;
else
    is_running = 0;
    timer = 0;
end

%% ===== 功率选择 =====
if P_target <= 0
    P_out = 0;
elseif timer <= T_warmup
    % 30分钟内，限制最大5kW
    P_out = min(P_target, P_warmup);
else
    % 30分钟后，输出等于输入
    P_out = P_target;
end

end

== matlab function Energy/240kW功率分配-3挡位分配64，128，256 ==
  data: V_battery input; SOC input; P_battery input; P1 output; P2 output; P3 output; P4 output; P5 output; P6 output; P7 output; P8 output; P_fuelcell input
function [P1, P2, P3, P4, P5, P6, P7, P8] = fcn(V_battery, SOC, P_battery, P_fuelcell)
%% 能量管理控制器 - 3挡位功率分配（带滞回+SOC保护）
%% 输入:
%%   SOC        - 蓄电池荷电状态 (0~1)
%%   P_battery  - 蓄电池功率 (kW)，放电为正，充电为负
%%   P_fuelcell - 燃料电池功率 (kW)
%%   V_battery  - 蓄电池电压 (V)
%% 输出:
%%   P1~P8      - 8个通道功率分配 (kW)

%% ===== SOC安全区间 =====
SOC_high = 0.8;   % SOC上限
SOC_low = 0.5;    % SOC下限

%% ===== SOC充放电滞回 =====
SOC_charge_start = 0.5;
SOC_charge_stop = 0.7;
SOC_discharge_start = 0.8;
SOC_discharge_stop = 0.6;

%% ===== 挡位滞回阈值 (kW) =====
Gear_1_to_2_up = 100;
Gear_2_to_1_down = 80;
Gear_2_to_3_up = 200;
Gear_3_to_2_down = 160;

%% ===== 过载阈值 =====
P_overload = 300;
P_max_each = 32;

%% ===== 充放电电流 =====
I_charge = 100;

%% ===== 滞回控制状态 =====
persistent charge_mode discharge_mode gear_state
if isempty(charge_mode)
    charge_mode = 0;
    discharge_mode = 0;
    gear_state = 1;
end

%% ===== SOC滞回控制逻辑 =====
if SOC < SOC_charge_start
    charge_mode = 1;
elseif SOC >= SOC_charge_stop
    charge_mode = 0;
end

if SOC > SOC_discharge_start
    discharge_mode = 1;
elseif SOC <= SOC_discharge_stop
    discharge_mode = 0;
end

%% ===== 计算系统需求功率 (kW) =====
P_base = P_fuelcell + P_battery;

if charge_mode == 1
    P_demand = P_base + V_battery * I_charge / 1000;
elseif discharge_mode == 1
    P_demand = P_base - V_battery * I_charge / 1000;
else
    P_demand = P_base;
end

P_demand = max(0, P_demand);

%% ===== 过载保护 =====
if P_base > P_overload
    P1 = P_max_each; P2 = P_max_each; P3 = P_max_each; P4 = P_max_each;
    P5 = 0; P6 = 0; P7 = 0; P8 = 0;
else
    %% ===== 挡位滞回切换逻辑 =====
    if gear_state == 1
        if P_demand > Gear_1_to_2_up
            gear_state = 2;
        end
    elseif gear_state == 2
        if P_demand < Gear_2_to_1_down
            gear_state = 1;
        elseif P_demand > Gear_2_to_3_up
            gear_state = 3;
        end
    else
        if P_demand < Gear_3_to_2_down
            gear_state = 2;
        end
    end
    
    %% ===== SOC保护：强制调整挡位 =====
    % SOC > 0.8 且蓄电池仍在充电（P_battery < 0），强制降挡
    if SOC > SOC_high && P_battery < 0
        if gear_state > 1
            gear_state = gear_state - 1;
        end
    end
    
    % SOC < 0.5 且蓄电池仍在放电（P_battery > 0），强制升挡
    if SOC < SOC_low && P_battery > 0
        if gear_state < 3
            gear_state = gear_state + 1;
        end
    end
    
    %% ===== 按挡位分配功率 =====
    if gear_state == 1
        % 挡位1: 64kW
        P1 = 16; P2 = 16; P3 = 16; P4 = 16;
        P5 = 0; P6 = 0; P7 = 0; P8 = 0;
    elseif gear_state == 2
        % 挡位2: 128kW
        P1 = 32; P2 = 32; P3 = 32; P4 = 32;
        P5 = 0; P6 = 0; P7 = 0; P8 = 0;
    else
        % 挡位3: 256kW
        P1 = 32; P2 = 32; P3 = 32; P4 = 32;
        P5 = 32; P6 = 32; P7 = 32; P8 = 32;
    end
end

end

== matlab function Energy/工况1 ==
  data: t input; P_out output
function P_out = fcn(t)
%% 工况生成函数（末尾添加0kW停机段）
%% 输入: t - 仿真时间 (s)
%% 输出: P_out - 功率 (kW)

%% ===== 工况数据 =====
% 功率点 (kW) - 末尾添加0
P_table = [64.039, 57.95, 72.892, 53.239, 371.17, 55.79, 55.814, 65.851, ...
           45.775, 69.748, 65.851, 45.775, 69.748, 65.851, 45.775, 81.182, ...
           57.663, 57.95, 64.502, 0];

% 持续时间 (h) - 末尾添加600s = 1/6小时
T_duration = [3, 72, 5, 36, 0.2, 12, 9, 4.2, 6.3, 3.5, 4.2, 6.3, 3.5, ...
              4.2, 6.3, 8, 4, 73, 3, 1/6] * 3600;

%% ===== 累计时间断点 =====
% 原949320 + 600 = 949920
T_bp = [0, 10800, 270000, 288000, 417600, 418320, 461520, 493920, 509040, ...
        531720, 544320, 559440, 582120, 594720, 609840, 632520, 661320, ...
        675720, 938520, 949320, 949920];

%% ===== 根据时间查找功率 =====
n = 20;  % 改为20
P_out = P_table(n);

for k = 1:n
    if t >= T_bp(k) && t < T_bp(k+1)
        P_out = P_table(k);
        break;
    end
end

end

== matlab function Energy/工况2 ==
  data: t input; P_out output
function P_out = fcn(t)
%% 工况生成函数2
%% 输入: t - 仿真时间 (s)
%% 输出: P_out - 功率 (kW)

%% ===== 工况数据 =====
% 功率点 (kW)
P_table = [64.039, 57.95, 72.892, 53.239, 371.167, 81.182, 152.606, ...
           55.814, 52.287, 87.468, 57.663, 57.95, 64.502];

% 持续时间 (s) = 小时 × 3600
T_duration = [3, 112, 5, 6, 0.2, 8, 8, 3, 0.3, 1, 4, 112, 3] * 3600;

%% ===== 累计时间断点 =====
T_bp = [0, 10800, 414000, 432000, 453600, 454320, 483120, 511920, ...
        522720, 523800, 527400, 541800, 945000, 955800];

%% ===== 根据时间查找功率 =====
n = 13;
P_out = P_table(n);  % 默认最后一个

for k = 1:n
    if t >= T_bp(k) && t < T_bp(k+1)
        P_out = P_table(k);
        break;
    end
end

end

== matlab function Energy/推进电机 ==
  data: t input; I_motor output
function I_motor = motor_startup_current(t)
%#codegen
% 电机启动电流曲线 - 直接影响母线电压
% 输入: t - 仿真时间(s)
% 输出: I_motor - 电机电流(A)
%
% 母线电压变化: ΔV = I_motor × R_int
% 这才是电机对母线的真正影响！

persistent time_data current_data

if isempty(time_data)
    % 时间 (秒，从0开始)
    time_data = [0; 5; 6; 7; 8; 9; 10; 11; 12; 13; 14; 15; 16; ...
                 20; 30; 41; 51; 61; 71; 77; 83; 91; 97; 106; ...
                 116; 136; 156; 176; 196; 216; 236; 256; 276; ...
                 296; 350; 400; 500; 600; 700; 834];
    
    % 电流 (A) - 原始数据"支路一输入电流"
    current_data = [0; 1.5; 3.4; 0.2; -0.2; 1.2; 0.4; 0; 0.3; ...
                    0.6; 0.2; 0.2; 0.5; 1.7; 9.3; 17.4; 41.8; ...
                    75.7; 104.6; 121.0; 138.4; 160.2; 173.9; 199.0; ...
                    223.1; 282.8; 305.1; 314.1; 320.6; 320.4; 320.3; ...
                    325.1; 314.5; 313.3; 333.2; 333.9; 341.7; 343.4; ...
                    342.0; 342.0];
end

% 插值获取当前电流
t_clamped = max(0, min(t, time_data(end)));
I_motor = interp1(time_data, current_data, t_clamped, 'linear', 0);
I_motor = max(0, I_motor);

end

== matlab function Energy/阀控式铅酸蓄电池1 ==
  data: SOC_init input; dt input; V output; I_pack input; SOC output
function [V, SOC] = fcn(SOC_init,dt,I_pack)
%% VRLA电池组二阶RC模型 - 231串2并
%% 输入: I_pack - 电池组电流(A), 放电为正
%% 输出: V - 电池组电压(V), SOC - 荷电状态(0~1)

%% ===== 电池组配置 =====
N_series = 231;    % 串联数量
N_parallel = 2;    % 并联数量

%% ===== 单体参数 =====
Q_10h = 1025.0000;
k_peukert = 1.273470;
SOC_bp = [1.00, 0.90, 0.80, 0.70, 0.60, 0.50, 0.40, 0.30, 0.20, 0.10, 0.05, 0.00];
OCV_table = [2.1500, 2.1271, 2.1077, 2.0929, 2.0783, 2.0600, 2.0384, 2.0107, 1.9800, 1.9502, 1.9352, 1.9200];
R0_table = [0.000258, 0.000258, 0.000258, 0.000258, 0.000258, 0.000258, 0.000258, 0.000258, 0.000258, 0.000260, 0.000262, 0.000268];
R1_table = [0.000020, 0.000020, 0.000020, 0.000020, 0.000020, 0.000020, 0.000020, 0.000022, 0.000030, 0.000065, 0.000114, 0.000220];
R2_table = [0.000080, 0.000080, 0.000080, 0.000080, 0.000080, 0.000080, 0.000082, 0.000089, 0.000120, 0.000259, 0.000458, 0.000880];
tau1 = 150.0000;
tau2 = 1250.0889;
alpha = 0.300000;

%% ===== 并联分流：计算单体电流 =====
I = I_pack / N_parallel;

%% ===== 模型计算(勿改) =====
persistent SOC_s V1 V2 flag
if isempty(flag), SOC_s=SOC_init; V1=0; V2=0; flag=1; end
s = max(0.001, min(1, SOC_s));
Ia = max(abs(I), 0.1);
Qe = Q_10h * (100/Ia)^(k_peukert-1);

%% 初始化变量
OCV = OCV_table(1); R0 = R0_table(1); R1b = R1_table(1); R2b = R2_table(1);

%% 线性插值
n = 12;
for k=1:n-1
    if s<=SOC_bp(k) && s>=SOC_bp(k+1)
        t=(s-SOC_bp(k+1))/(SOC_bp(k)-SOC_bp(k+1));
        OCV=OCV_table(k+1)+t*(OCV_table(k)-OCV_table(k+1));
        R0=R0_table(k+1)+t*(R0_table(k)-R0_table(k+1));
        R1b=R1_table(k+1)+t*(R1_table(k)-R1_table(k+1));
        R2b=R2_table(k+1)+t*(R2_table(k)-R2_table(k+1));
        break;
    end
end

If = (Ia/100)^(alpha-1);
R1 = R1b*If; R2 = R2b*If;
e1=exp(-dt/tau1); e2=exp(-dt/tau2);
V1=V1*e1+I*R1*(1-e1);
V2=V2*e2+I*R2*(1-e2);

%% ===== 单体电压 =====
V_cell = OCV - I*R0 - V1 - V2;
V_cell = max(1.6, min(2.4, V_cell));

%% ===== 串联：电池组电压 =====
V = N_series * V_cell;

%% ===== SOC更新 =====
SOC_s = max(0, min(1, s - I*dt/(3600*Qe)));
SOC = SOC_s;
end

== matlab function Energy/Subsystem1/DCDC1_2 ==
  data: V_out input; I_in input; V_in input; I_out output
function I_out = fcn(V_out,I_in, V_in)
%% DCDC模型 - 输入电流计算输出电流
%% 输入:
%%   I_in  - 输入电流 (A)
%%   V_in  - 输入电压 (V)
%%   V_out - 输出电压 (V)
%% 输出:
%%   I_out - 输出电流 (A)

%% ===== 效率MAP表 =====
% 输入电压断点 (V)
V_bp = [160, 180, 200, 220, 240, 260, 280];

% 输入电流断点 (A)
I_bp = [0, 20, 40, 60, 80, 100, 120, 140, 160, 180, 200];

% 效率表 (%)，行=电流，列=电压
Eta_map = [
    86, 86, 86, 86, 86, 86, 86;
    88, 88, 87, 87, 87, 87, 86;
    92, 91, 91, 90, 89, 88, 87;
    94, 93, 93, 92, 91, 90, 88;
    94.5, 94, 94, 93, 92, 91, 89;
    95, 94.5, 94, 93.5, 93, 91, 90;
    95, 94.5, 94.5, 94, 93, 92, 91;
    95, 95, 94.5, 94, 93.5, 93, 91;
    95, 95, 94.5, 94, 93, 92, 91;
    95, 94.5, 94.5, 93, 92, 91, 91;
    95, 94.5, 94, 92, 91, 91, 91
] / 100;

%% ===== 输入限幅 =====
V_in_clamp = max(160, min(280, V_in));
I_in_clamp = max(0, min(200, I_in));

%% ===== 查表获取效率 =====
% 找电压区间
nV = 7;
jV = 1;
for j = 1:nV-1
    if V_in_clamp >= V_bp(j) && V_in_clamp <= V_bp(j+1)
        jV = j;
        break;
    end
end
if V_in_clamp >= V_bp(nV)
    jV = nV - 1;
end
tV = (V_in_clamp - V_bp(jV)) / (V_bp(jV+1) - V_bp(jV));

% 找电流区间
nI = 11;
iI = 1;
for i = 1:nI-1
    if I_in_clamp >= I_bp(i) && I_in_clamp <= I_bp(i+1)
        iI = i;
        break;
    end
end
if I_in_clamp >= I_bp(nI)
    iI = nI - 1;
end
tI = (I_in_clamp - I_bp(iI)) / (I_bp(iI+1) - I_bp(iI));

% 双线性插值
eta_11 = Eta_map(iI, jV);
eta_12 = Eta_map(iI, jV+1);
eta_21 = Eta_map(iI+1, jV);
eta_22 = Eta_map(iI+1, jV+1);

eta_1 = eta_11 + tV * (eta_12 - eta_11);
eta_2 = eta_21 + tV * (eta_22 - eta_21);
eta = eta_1 + tI * (eta_2 - eta_1);

%% ===== 计算输出电流 =====
P_in = V_in * I_in;
P_out = P_in * eta;
V_out_safe = max(V_out, 1);
I_out = P_out / V_out_safe;

end

== matlab function Energy/Subsystem1/目标输出功率 ==
  data: P_target input; dt input; P_out output
function P_out = fcn(P_target, dt)
%% 燃料电池预热控制器 - 带热机跳过功能
%% 输入:
%%   P_target - 目标功率 (kW)
%%   dt       - 采样时间 (s)
%% 输出:
%%   P_out    - 输出功率 (kW)

%% ===== 参数设置 =====
T_warmup = 1800;       % 预热时间 30分钟
P_warmup = 5;          % 预热功率上限 5kW
T_hot_keep = 18000;    % 热机保持时间 5小时 = 5*3600s

%% ===== 状态变量 =====
persistent timer_run timer_stop is_running is_hot
if isempty(timer_run)
    timer_run = 0;      % 运行计时器
    timer_stop = 0;     % 停机计时器
    is_running = 0;     % 运行状态
    is_hot = 0;         % 热机状态：0=冷机，1=已热机
end

%% ===== 状态机逻辑 =====
if P_target > 0
    % 启动/运行中
    if is_running == 0
        % 刚启动
        is_running = 1;
        timer_run = 0;
        
        % 判断是否需要热机
        if is_hot == 1 && timer_stop <= T_hot_keep
            % 停机5小时内，跳过热机
            timer_run = T_warmup + 1;  % 直接跳过热机阶段
        else
            % 冷机或停机超过5小时，需要热机
            timer_run = 0;
        end
    end
    
    timer_run = timer_run + dt;
    timer_stop = 0;  % 清空停机计时
    
    % 完成热机后标记
    if timer_run > T_warmup
        is_hot = 1;
    end
else
    % 停机
    if is_running == 1
        % 刚停机
        is_running = 0;
        timer_stop = 0;
    end
    
    timer_stop = timer_stop + dt;
    timer_run = 0;
    
    % 停机超过5小时，热机状态清除
    if timer_stop > T_hot_keep
        is_hot = 0;
    end
end

%% ===== 功率选择 =====
if P_target <= 0
    P_out = 0;
elseif timer_run <= T_warmup
    % 热机阶段，限制最大5kW
    P_out = min(P_target, P_warmup);
else
    % 热机完成，输出等于输入
    P_out = P_target;
end

end

== matlab function Energy/Subsystem1/输出电流加载限制 ==
  data: I_target input; I_current input; I_out output; dt input
function I_out = fcn(I_target,I_current,  dt)
%% 电流斜坡控制器 - 反馈版
%% 输入:
%%   I_current - 当前电流 (A)，从输出反馈
%%   I_target  - 目标电流 (A) 
%%   dt        - 采样时间 (s)
%% 输出:
%%   I_out     - 输出电流 (A)

%% ===== 参数设置 =====
rate_up = 1;    % 上升速率 1A/s
rate_down = 2;  % 下降速率 2A/s

%% ===== 斜坡控制 =====
delta = I_target - I_current;

if delta > 0
    % 目标 > 当前，每秒+1A
    I_out = I_current + rate_up * dt;
    if I_out > I_target
        I_out = I_target;
    end
elseif delta < 0
    % 目标 < 当前，每秒-2A
    I_out = I_current - rate_down * dt;
    if I_out < I_target
        I_out = I_target;
    end
else
    I_out = I_current;
end

%% ===== 输出限幅 =====
I_out = max(0, I_out);

end

== matlab function Energy/Subsystem2/32kW燃料电池 ==
  data: I_in input; V output
function V = fcn(I_in)
%% 燃料电池模型 - 极化曲线
%% 输入: I_in - 输入电流 (A)
%% 输出: V    - 输出电压 (V)

%% ===== 极化曲线数据 =====
I_table = [0, 16.77, 31.67, 48.13, 64.92, 80.76, 98.06, 115.48, 132.58, 150.51, 170.44, 186.07];
V_table = [248.1, 218.42, 212.82, 207.8, 205, 202.68, 200, 197.8, 196.44, 194.26, 192.66, 191.2];

%% ===== 电流限幅 =====
I_max = 186.07;
I = max(0, min(I_in, I_max));

%% ===== 根据电流查找电压 =====
V = V_table(1);  % 初始化
n = 12;

for k = 1:n-1
    if I >= I_table(k) && I <= I_table(k+1)
        t = (I - I_table(k)) / (I_table(k+1) - I_table(k));
        V = V_table(k) + t * (V_table(k+1) - V_table(k));
        break;
    end
end

if I >= I_table(n)
    V = V_table(n);
end

end

== matlab function Energy/Subsystem2/DCDC1_1 ==
  data: P_out input; V_out input; I_out output; V_in input; I_in output
function [I_out, I_in] = fcn(P_out, V_out, V_in)
%% DCDC模型 - 输出功率反算输入电流
%% 输入:
%%   P_out - 输出功率 (W)
%%   V_out - 输出电压 (V)
%%   V_in  - 输入电压 (V)
%% 输出:
%%   I_out - 输出电流 (A)
%%   I_in  - 输入电流 (A)

%% ===== 效率MAP表 =====
% 输入电压断点 (V)
V_bp = [160, 180, 200, 220, 240, 260, 280];

% 输入电流断点 (A)
I_bp = [0, 20, 40, 60, 80, 100, 120, 140, 160, 180, 200];

% 效率表 (%)，行=电流，列=电压
Eta_map = [
    86, 86, 86, 86, 86, 86, 86;
    88, 88, 87, 87, 87, 87, 86;
    92, 91, 91, 90, 89, 88, 87;
    94, 93, 93, 92, 91, 90, 88;
    94.5, 94, 94, 93, 92, 91, 89;
    95, 94.5, 94, 93.5, 93, 91, 90;
    95, 94.5, 94.5, 94, 93, 92, 91;
    95, 95, 94.5, 94, 93.5, 93, 91;
    95, 95, 94.5, 94, 93, 92, 91;
    95, 94.5, 94.5, 93, 92, 91, 91;
    95, 94.5, 94, 92, 91, 91, 91
] / 100;

%% ===== 输出电流（直接计算） =====
V_out_safe = max(V_out, 1);
I_out = 1000*P_out / V_out_safe;

%% ===== 迭代求输入电流 =====
V_in_clamp = max(160, min(280, V_in));
V_in_safe = max(V_in, 1);

% 初始估计效率
eta = 0.94;

% 迭代3次足够收敛
for iter = 1:3
    % 根据效率计算输入功率和电流
    P_in = 1000*P_out / eta;
    I_in_est = P_in / V_in_safe;
    I_in_clamp = max(0, min(200, I_in_est));
    
    % 查表获取新效率
    eta = lookup_eta(V_in_clamp, I_in_clamp, V_bp, I_bp, Eta_map);
end

%% ===== 最终输入电流 =====
P_in = 1000*P_out / eta;
I_in = P_in / V_in_safe;

end

%% ===== 效率查表函数 =====
function eta = lookup_eta(V_in, I_in, V_bp, I_bp, Eta_map)
    % 找电压区间
    nV = 7;
    jV = 1;
    for j = 1:nV-1
        if V_in >= V_bp(j) && V_in <= V_bp(j+1)
            jV = j;
            break;
        end
    end
    if V_in >= V_bp(nV)
        jV = nV - 1;
    end
    tV = (V_in - V_bp(jV)) / (V_bp(jV+1) - V_bp(jV));
    
    % 找电流区间
    nI = 11;
    iI = 1;
    for i = 1:nI-1
        if I_in >= I_bp(i) && I_in <= I_bp(i+1)
            iI = i;
            break;
        end
    end
    if I_in >= I_bp(nI)
        iI = nI - 1;
    end
    tI = (I_in - I_bp(iI)) / (I_bp(iI+1) - I_bp(iI));
    
    % 双线性插值
    eta_11 = Eta_map(iI, jV);
    eta_12 = Eta_map(iI, jV+1);
    eta_21 = Eta_map(iI+1, jV);
    eta_22 = Eta_map(iI+1, jV+1);
    
    eta_1 = eta_11 + tV * (eta_12 - eta_11);
    eta_2 = eta_21 + tV * (eta_22 - eta_21);
    eta = eta_1 + tI * (eta_2 - eta_1);
end
